simulink model "UWAFT_Blazer_P4_4WD_Opt"  (R2023b)
settings: Solver=VariableStepAuto  StartTime=0.0  StopTime=inf  RelTol=1e-3
StopFcn:
  | clear send_to_vecu
libraries: simulink x1
settings Model: Creator=Admin  LastModifiedBy=Admin

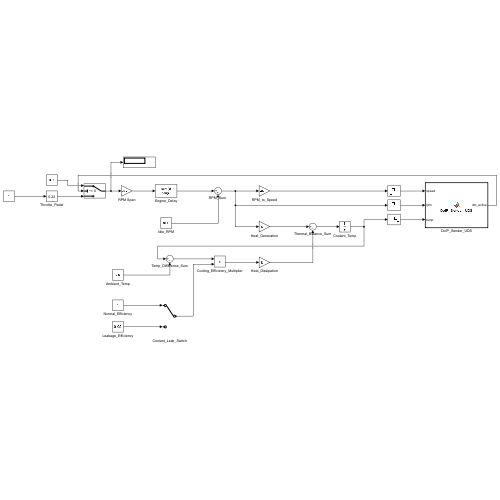
[thumbnail: Simulink's stored preview of the top-level diagram]
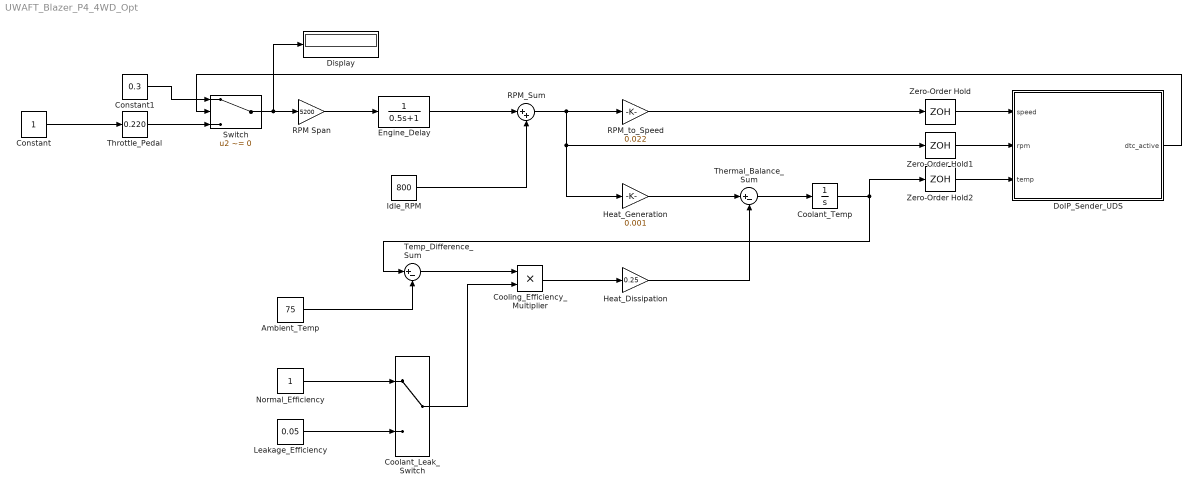
== system UWAFT_Blazer_P4_4WD_Opt ==
  Ambient_Temp : Constant  Value=75
  Constant : Constant
  Constant1 : Constant  Value=0.3
  Coolant_Leak_Switch : ManualSwitch
  Coolant_Temp : Integrator  InitialCondition=90
  Cooling_Efficiency_Multiplier : Product
  Display : Display
  DoIP_Sender_UDS : MATLAB Function  TreatAsAtomicUnit=on  SystemSampleTime=0.1
  Engine_Delay : TransferFcn  Denominator=[0.5 1]
  Heat_Dissipation : Gain  Gain=0.25
  Heat_Generation : Gain  Gain=0.001
  Idle_RPM : Constant  Value=800
  Leakage_Efficiency : Constant  Value=0.05
  Normal_Efficiency : Constant
  RPM Span : Gain  Gain=5200
  "RPM_Sum " : Sum  Inputs=|++
  RPM_to_Speed : Gain  Gain=0.022
  Switch : Switch  Criteria=u2 ~= 0  SaturateOnIntegerOverflow=off  InputSameDT=off
  Temp_Difference_Sum : Sum  Inputs=|+-
  Thermal_Balance_Sum : Sum  Inputs=|+-
  Throttle_Pedal : simulink/Math Operations/Slider Gain  gain=0.220  low=0  high=1
  Zero-Order Hold : ZeroOrderHold  SampleTime=0.1
  Zero-Order Hold1 : ZeroOrderHold  SampleTime=0.1
  Zero-Order Hold2 : ZeroOrderHold  SampleTime=0.1
  wires:
  RPM Span/1 -> Engine_Delay/1
  Engine_Delay/1 -> "RPM_Sum "/1
  Idle_RPM/1 -> "RPM_Sum "/2
  "RPM_Sum "/1 -> Heat_Generation/1, Zero-Order Hold1/1, RPM_to_Speed/1
  Heat_Generation/1 -> Thermal_Balance_Sum/1
  Coolant_Temp/1 -> Zero-Order Hold2/1, Temp_Difference_Sum/1
  Temp_Difference_Sum/1 -> Cooling_Efficiency_Multiplier/1
  Normal_Efficiency/1 -> Coolant_Leak_Switch/1
  Leakage_Efficiency/1 -> Coolant_Leak_Switch/2
  Coolant_Leak_Switch/1 -> Cooling_Efficiency_Multiplier/2
  Cooling_Efficiency_Multiplier/1 -> Heat_Dissipation/1
  Heat_Dissipation/1 -> Thermal_Balance_Sum/2
  Thermal_Balance_Sum/1 -> Coolant_Temp/1
  RPM_to_Speed/1 -> Zero-Order Hold/1
  Ambient_Temp/1 -> Temp_Difference_Sum/2
  Constant/1 -> Throttle_Pedal/1
  Switch/1 -> Display/1, RPM Span/1
  Constant1/1 -> Switch/1
  DoIP_Sender_UDS/1(dtc_active) -> Switch/2
  Throttle_Pedal/1 -> Switch/3
  Zero-Order Hold/1 -> DoIP_Sender_UDS/1(speed)
  Zero-Order Hold2/1 -> DoIP_Sender_UDS/3(temp)
  Zero-Order Hold1/1 -> DoIP_Sender_UDS/2(rpm)

== matlab function UWAFT_Blazer_P4_4WD_Opt/DoIP_Sender_UDS ==
  settings: updateMethod=DISCRETE
  data: speed input; dtc_active output; rpm input; temp input
function dtc_active = DoIP_Sender_UDS(speed, rpm, temp)
    coder.extrinsic('send_to_vecu');
    dtc_active = double(0); % Khởi tạo biến đầu ra
    dtc_active = send_to_vecu(speed, rpm, temp);
end
